simulink model "SYDE_351_Project"  (R2022b)
settings: Solver=VariableStepAuto  StartTime=0.0  StopTime=23.55  RelTol=1e-3
values from neighbouring files (symbols this model uses):
  d = 2.5e-2    (= 0.025)    [SYDE_351_Project_Parameters.m]
  J = (1/2)*(M * (R_cyl)^2)    (= 0.625)    [SYDE_351_Project_Parameters.m]
  K_b = 0.3247    [SYDE_351_Project_Parameters.m]
  K_t = 0.3248    [SYDE_351_Project_Parameters.m]
  L = 25e-2    (= 0.25)    [SYDE_351_Project_Parameters.m]
  L_a = 6.6e-3    (= 0.0066)    [SYDE_351_Project_Parameters.m]
  M = 20    [SYDE_351_Project_Parameters.m]
  N = 1    [SYDE_351_Project_Parameters.m]
  R = 5e-2    (= 0.05)    [SYDE_351_Project_Parameters.m]
  R_a = 4    [SYDE_351_Project_Parameters.m]
libraries: slpidlib x6
settings Model: Creator=danielkang  LastModifiedBy=danielkang

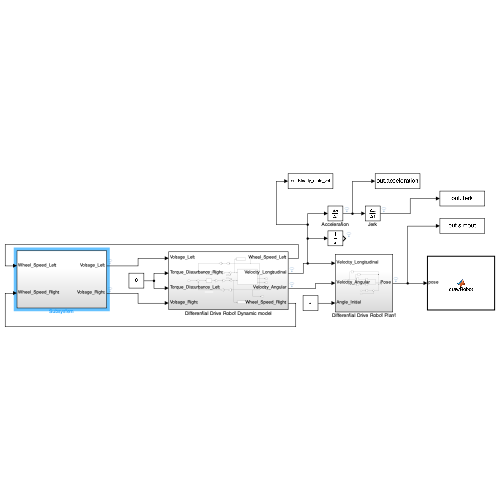
[thumbnail: Simulink's stored preview of the top-level diagram]
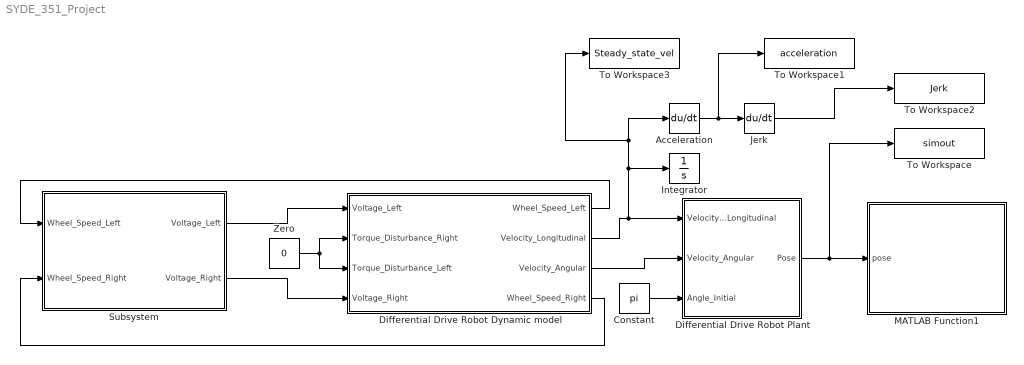
== system SYDE_351_Project ==
  Acceleration : Derivative
  Constant : Constant  Value=pi
  Differential Drive Robot Dynamic model : Subsystem
  Differential Drive Robot Plant : Subsystem
  Integrator : Integrator
  Jerk : Derivative
  MATLAB Function1 : MATLAB Function  TreatAsAtomicUnit=on
  Subsystem : Subsystem
  To Workspace : ToWorkspace  VariableName=simout  SampleTime=-1
      settings: Save2DSignal=2-D array (concatenate along first dimension)
  To Workspace1 : ToWorkspace  VariableName=acceleration  SampleTime=-1
      settings: Save2DSignal=2-D array (concatenate along first dimension)
  To Workspace2 : ToWorkspace  VariableName=Jerk  SampleTime=-1
      settings: Save2DSignal=2-D array (concatenate along first dimension)
  To Workspace3 : ToWorkspace  VariableName=Steady_state_vel  SampleTime=-1
      settings: Save2DSignal=2-D array (concatenate along first dimension)
  Zero : Constant  Value=0  OutDataTypeStr=Inherit: Inherit via back propagation
  wires:
  Zero/1 -> Differential Drive Robot Dynamic model/3(Torque_Disturbance_Left), Differential Drive Robot Dynamic model/2(Torque_Disturbance_Right)
  Differential Drive Robot Dynamic model/3(Velocity_Angular) -> Differential Drive Robot Plant/2(Velocity_Angular)
  Differential Drive Robot Plant/1(Pose) -> To Workspace/1, MATLAB Function1/1(pose)
  Differential Drive Robot Dynamic model/2(Velocity_Longitudinal) -> Integrator/1, To Workspace3/1, Acceleration/1, Differential Drive Robot Plant/1(Velocity_Longitudinal)
  Constant/1 -> Differential Drive Robot Plant/3(Angle_Initial)
  Acceleration/1 -> To Workspace1/1, Jerk/1
  Jerk/1 -> To Workspace2/1
  Subsystem/1(Voltage_Left) -> Differential Drive Robot Dynamic model/1(Voltage_Left)
  Subsystem/2(Voltage_Right) -> Differential Drive Robot Dynamic model/4(Voltage_Right)
  Differential Drive Robot Dynamic model/1(Wheel_Speed_Left) -> Subsystem/1(Wheel_Speed_Left)
  Differential Drive Robot Dynamic model/4(Wheel_Speed_Right) -> Subsystem/2(Wheel_Speed_Right)

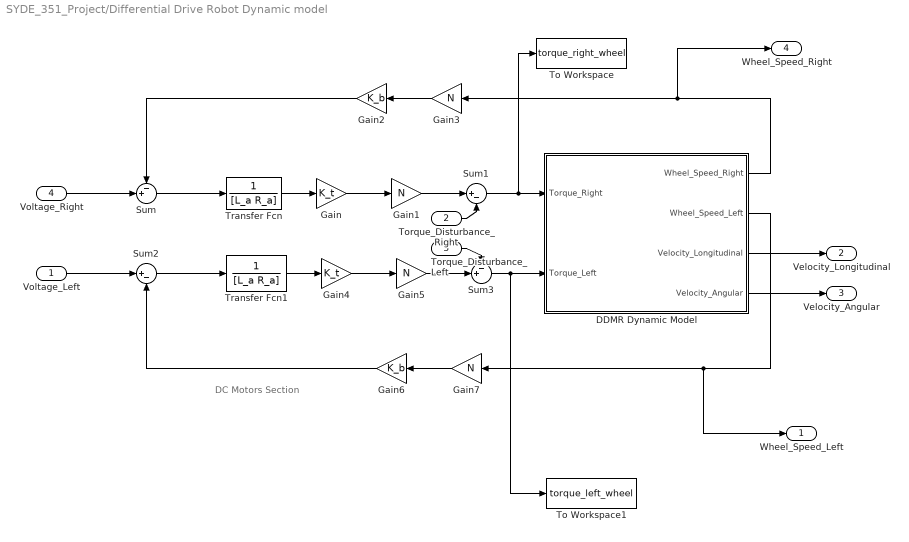
== system SYDE_351_Project/Differential Drive Robot Dynamic model ==
  note: DC Motors Section
  Voltage_Left : Inport
  Torque_Disturbance_Right : Inport  Port=2
  Torque_Disturbance_Left : Inport  Port=3
  Voltage_Right : Inport  Port=4
  DDMR Dynamic Model : Subsystem
  Gain : Gain  Gain=K_t
  Gain{1,3,5,7} (4 alike) : Gain  Gain=N
  Gain2 : Gain  Gain=K_b
  Gain4 : Gain  Gain=K_t
  Gain6 : Gain  Gain=K_b
  Sum : Sum  Inputs=-+|
  Sum1 : Sum  Inputs=|+-
  Sum2 : Sum  Inputs=|+-
  Sum3 : Sum  Inputs=-+|
  To Workspace : ToWorkspace  VariableName=torque_right_wheel  SaveFormat=Structure With Time  SampleTime=-1
      settings: Save2DSignal=2-D array (concatenate along first dimension)
  To Workspace1 : ToWorkspace  VariableName=torque_left_wheel  SaveFormat=Structure With Time  SampleTime=-1
  Transfer Fcn : TransferFcn  Denominator=[L_a R_a]
  Transfer Fcn1 : TransferFcn  Denominator=[L_a R_a]
  Wheel_Speed_Left : Outport
  Velocity_Longitudinal : Outport  Port=2
  Velocity_Angular : Outport  Port=3
  Wheel_Speed_Right : Outport  Port=4
  wires:
  Torque_Disturbance_Left/1 -> Sum3/1
  Gain5/1 -> Sum3/2
  Torque_Disturbance_Right/1 -> Sum1/2
  Gain7/1 -> Gain6/1
  Sum/1 -> Transfer Fcn/1
  Transfer Fcn1/1 -> Gain4/1
  Sum3/1 -> To Workspace1/1, DDMR Dynamic Model/2(Torque_Left)
  Sum1/1 -> To Workspace/1, DDMR Dynamic Model/1(Torque_Right)
  Gain6/1 -> Sum2/2
  Gain3/1 -> Gain2/1
  Sum2/1 -> Transfer Fcn1/1
  Gain4/1 -> Gain5/1
  Voltage_Right/1 -> Sum/2
  Voltage_Left/1 -> Sum2/1
  Gain2/1 -> Sum/1
  Transfer Fcn/1 -> Gain/1
  Gain/1 -> Gain1/1
  Gain1/1 -> Sum1/1
  DDMR Dynamic Model/1(Wheel_Speed_Right) -> Wheel_Speed_Right/1, Gain3/1
  DDMR Dynamic Model/3(Velocity_Longitudinal) -> Velocity_Longitudinal/1
  DDMR Dynamic Model/4(Velocity_Angular) -> Velocity_Angular/1
  DDMR Dynamic Model/2(Wheel_Speed_Left) -> Wheel_Speed_Left/1, Gain7/1

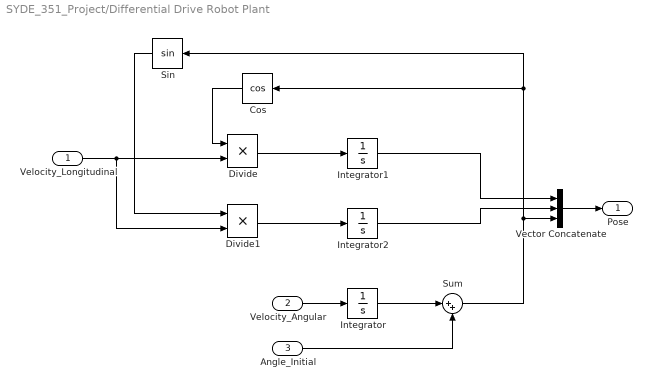
== system SYDE_351_Project/Differential Drive Robot Plant ==
  Velocity_Longitudinal : Inport
  Velocity_Angular : Inport  Port=2
  Angle_Initial : Inport  Port=3
  Cos : Trigonometry  Operator=cos
  Divide : Product  Inputs=**
  Divide1 : Product  Inputs=**
  Integrator : Integrator
  Integrator1 : Integrator
  Integrator2 : Integrator
  Sin : Trigonometry
  Sum : Sum  Inputs=|++
  Vector Concatenate : Concatenate  NumInputs=3
  Pose : Outport
  wires:
  Velocity_Angular/1 -> Integrator/1
  Cos/1 -> Divide/1
  Divide/1 -> Integrator1/1
  Integrator1/1 -> Vector Concatenate/1
  Velocity_Longitudinal/1 -> Divide1/2, Divide/2
  Divide1/1 -> Integrator2/1
  Integrator2/1 -> Vector Concatenate/2
  Sin/1 -> Divide1/1
  Vector Concatenate/1 -> Pose/1
  Angle_Initial/1 -> Sum/2
  Integrator/1 -> Sum/1
  Sum/1 -> Cos/1, Sin/1, Vector Concatenate/3

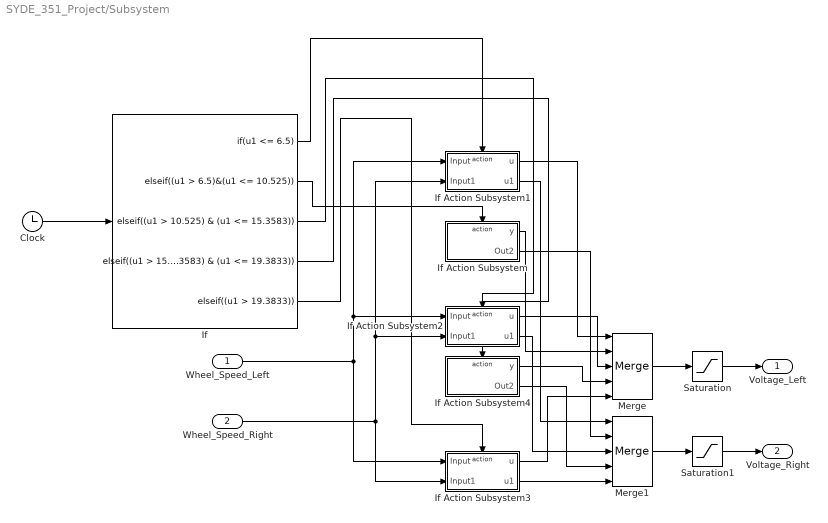
== system SYDE_351_Project/Subsystem ==
  Wheel_Speed_Left : Inport
  Wheel_Speed_Right : Inport  Port=2
  Clock : Clock
  If : If  IfExpression=u1 <= 6.5  ElseIfExpressions=(u1 > 6.5)&(u1 <= 10.525), (u1 > 10.525) & (u1 <= 15.3583), (u1 > 15.3583) & (u1 <= 19.3833),(u1 > 19.3833)  ShowElse=off
  If Action Subsystem : Subsystem  TreatAsAtomicUnit=on
  If Action Subsystem1 : Subsystem  TreatAsAtomicUnit=on
  If Action Subsystem2 : Subsystem  TreatAsAtomicUnit=on
  If Action Subsystem3 : Subsystem  TreatAsAtomicUnit=on
  If Action Subsystem4 : Subsystem  TreatAsAtomicUnit=on
  Merge : Merge  Inputs=5
  Merge1 : Merge  Inputs=5
  Saturation : Saturate  UpperLimit=500  LowerLimit=-500
  Saturation1 : Saturate  UpperLimit=500  LowerLimit=-500
  Voltage_Left : Outport
  Voltage_Right : Outport  Port=2
  wires:
  If Action Subsystem2/2(u1) -> Merge1/3
  If Action Subsystem2/1(u) -> Merge/3
  If Action Subsystem1/1(u) -> Merge/1
  If/1 -> If Action Subsystem1/Action
  If Action Subsystem1/2(u1) -> Merge1/1
  Clock/1 -> If/1
  Wheel_Speed_Left/1 -> If Action Subsystem1/1(Input), If Action Subsystem2/1(Input), If Action Subsystem3/1(Input)
  Wheel_Speed_Right/1 -> If Action Subsystem1/2(Input1), If Action Subsystem2/2(Input1), If Action Subsystem3/2(Input1)
  If/2 -> If Action Subsystem/Action
  If Action Subsystem/1(y) -> Merge/2
  If Action Subsystem/2(Out2) -> Merge1/2
  If/3 -> If Action Subsystem2/Action
  Saturation/1 -> Voltage_Left/1
  Merge/1 -> Saturation/1
  Merge1/1 -> Saturation1/1
  Saturation1/1 -> Voltage_Right/1
  If/4 -> If Action Subsystem4/Action
  If/5 -> If Action Subsystem3/Action
  If Action Subsystem4/1(y) -> Merge/4
  If Action Subsystem4/2(Out2) -> Merge1/4
  If Action Subsystem3/1(u) -> Merge/5
  If Action Subsystem3/2(u1) -> Merge1/5

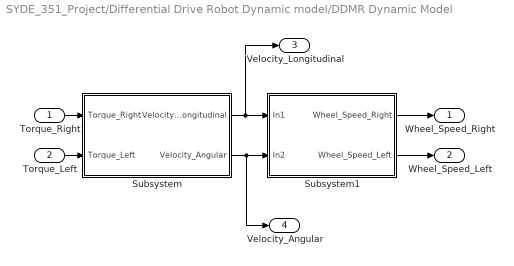
== system SYDE_351_Project/Differential Drive Robot Dynamic model/DDMR Dynamic Model ==
  Torque_Right : Inport
  Torque_Left : Inport  Port=2
  Subsystem : Subsystem
  Subsystem1 : Subsystem
  Wheel_Speed_Right : Outport
  Wheel_Speed_Left : Outport  Port=2
  Velocity_Longitudinal : Outport  Port=3
  Velocity_Angular : Outport  Port=4
  wires:
  Torque_Right/1 -> Subsystem/1(Torque_Right)
  Subsystem/1(Velocity_Longitudinal) -> Velocity_Longitudinal/1, Subsystem1/1(In1)
  Subsystem1/1(Wheel_Speed_Right) -> Wheel_Speed_Right/1
  Subsystem1/2(Wheel_Speed_Left) -> Wheel_Speed_Left/1
  Torque_Left/1 -> Subsystem/2(Torque_Left)
  Subsystem/2(Velocity_Angular) -> Velocity_Angular/1, Subsystem1/2(In2)

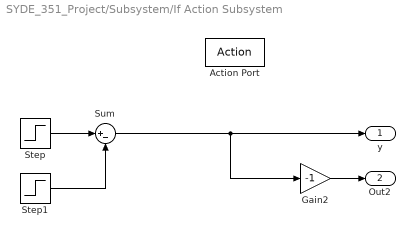
== system SYDE_351_Project/Subsystem/If Action Subsystem ==
  Action Port : ActionPort  ActionPortLabel=elseif((u1 > 6.5)&(u1 <= 10.525))
  Gain2 : Gain  Gain=-1
  Step : Step  Time=6.5  After=2  SampleTime=0
  Step1 : Step  Time=7.77  After=2  SampleTime=0
  Sum : Sum  Inputs=|+-
  y : Outport
  Out2 : Outport  Port=2
  wires:
  Gain2/1 -> Out2/1
  Sum/1 -> y/1, Gain2/1
  Step/1 -> Sum/1
  Step1/1 -> Sum/2

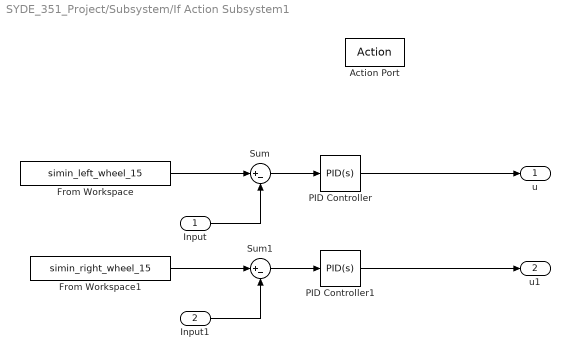
== system SYDE_351_Project/Subsystem/If Action Subsystem1 ==
  Input : Inport
  Input1 : Inport  Port=2
  Action Port : ActionPort  ActionPortLabel=if(u1 <= 6.5)
  From Workspace : FromWorkspace  VariableName=simin_left_wheel_15  ZeroCross=off
  From Workspace1 : FromWorkspace  VariableName=simin_right_wheel_15  ZeroCross=off
  PID Controller : slpidlib/PID Controller  Controller=PID  Form=Parallel  TimeDomain=Continuous-time  UseExternalTs=off  SampleTime=-1  IntegratorMethod=Forward Euler  FilterMethod=Forward Euler  ControllerParametersSource=internal  P=50  I=0  UseKiTs=off  D=0  N=100  UseFilter=on  TunerSelectOption=Transfer Function Based (PID Tuner App)  InitialConditionSource=internal  InitialConditionForIntegrator=0  InitialConditionForFilter=0  DifferentiatorICPrevScaledInput=0  ExternalReset=none  TrackingMode=off  Kt=1  LimitOutput=off  SatLimitsSource=internal  UpperSaturationLimit=inf  LowerSaturationLimit=-inf  LinearizeAsGain=on  AntiWindupMode=none  Kb=1  LimitIntegrator=off  UpperIntegratorSaturationLimit=inf  LowerIntegratorSaturationLimit=-inf  POutMin=[]  POutMax=[]  IOutMin=[]  IOutMax=[]  DOutMin=[]  DOutMax=[]  NOutMin=[]  NOutMax=[]  SumOutMin=[]  SumOutMax=[]  SaturationOutMin=[]  SaturationOutMax=[]  PParamMin=[]  PParamMax=[]  IParamMin=[]  IParamMax=[]  DParamMin=[]  DParamMax=[]  NParamMin=[]  NParamMax=[]  KbParamMin=[]  KbParamMax=[]  KtParamMin=[]  KtParamMax=[]  KbOutMin=[]  KbOutMax=[]  KtOutMin=[]  KtOutMax=[]  IntegratorOutMin=[]  IntegratorOutMax=[]  FilterOutMin=[]  FilterOutMax=[]  SumI1OutMin=[]  SumI1OutMax=[]  SumI2OutMin=[]  SumI2OutMax=[]  SumI3OutMin=[]  SumI3OutMax=[]  SumI4OutMin=[]  SumI4OutMax=[]  SumDOutMin=[]  SumDOutMax=[]  DifferentiatorOutMin=[]  DifferentiatorOutMax=[]  FilterDiffOutCoefMin=[]  FilterDiffOutCoefMax=[]  ReciprocalOutMin=[]  ReciprocalOutMax=[]  SumDenOutMin=[]  SumDenOutMax=[]  SumNumOutMin=[]  SumNumOutMax=[]  DivideOutMin=[]  DivideOutMax=[]  UdiffTsProdOutMin=[]  UdiffTsProdOutMax=[]  NTsProdOutMin=[]  NTsProdOutMax=[]  UintegralTsProdOutMin=[]  UintegralTsProdOutMax=[]  UngainTsProdOutMin=[]  UngainTsProdOutMax=[]  ClampingZeroOutDataTypeStr=Inherit: Inherit via back propagation  ClampingZeroOutMin=[]  ClampingZeroOutMax=[]  FilterDenConstantOutDataTypeStr=Inherit: Inherit via back propagation  FilterDenConstantOutMin=[]  FilterDenConstantOutMax=[]  PCopyOutDataTypeStr=Inherit: Inherit via back propagation  PCopyOutMin=[]  PCopyOutMax=[]  NCopyOutDataTypeStr=Inherit: Inherit via back propagation  NCopyOutMin=[]  NCopyOutMax=[]  IntegratorContinuousStateAttributes=''  IntegratorStateMustResolveToSignalObject=off  IntegratorRTWStateStorageClass=Auto  FilterContinuousStateAttributes=''  FilterStateMustResolveToSignalObject=off  FilterRTWStateStorageClass=Auto  ParallelPVariant=InternalParameters  IdealPVariant=Disabled  IVariant=InternalParameters  DVariant=InternalParameters  IntegratorVariant=Continuous  SatVariant=Disabled  AWVariant=Passthrough  PCopyVariant=Disabled  TRVariant=Disabled  FdbkBlocksVariant=Forward  IdealPFdbkVariant=Disabled  SatFdbkVariant=Disabled  DerivativeFilterVariant=ContFilter  NVariant=InternalParameters  NCopyVariant=Disabled  FilterICVariant=InternalICsFilter  IntegratorICVariant=InternalICs  ExternalResetVariant=Disabled  TRSumVariant=Passthrough  SumFdbkVariant=Disabled  SumVariant=Sum_PID  TsampFilterVariant=InternalTs  TsampNgainVariant=Passthrough  TsampIntegralVariant=Passthrough  ExternalSaturationOutDataTypeStr=Inherit: Same as second input
  PID Controller1 : slpidlib/PID Controller  Controller=PID  Form=Parallel  TimeDomain=Continuous-time  UseExternalTs=off  SampleTime=-1  IntegratorMethod=Forward Euler  FilterMethod=Forward Euler  ControllerParametersSource=internal  P=50  I=0  UseKiTs=off  D=0  N=100  UseFilter=on  TunerSelectOption=Transfer Function Based (PID Tuner App)  InitialConditionSource=internal  InitialConditionForIntegrator=0  InitialConditionForFilter=0  DifferentiatorICPrevScaledInput=0  ExternalReset=none  TrackingMode=off  Kt=1  LimitOutput=off  SatLimitsSource=internal  UpperSaturationLimit=inf  LowerSaturationLimit=-inf  LinearizeAsGain=on  AntiWindupMode=none  Kb=1  LimitIntegrator=off  UpperIntegratorSaturationLimit=inf  LowerIntegratorSaturationLimit=-inf  POutMin=[]  POutMax=[]  IOutMin=[]  IOutMax=[]  DOutMin=[]  DOutMax=[]  NOutMin=[]  NOutMax=[]  SumOutMin=[]  SumOutMax=[]  SaturationOutMin=[]  SaturationOutMax=[]  PParamMin=[]  PParamMax=[]  IParamMin=[]  IParamMax=[]  DParamMin=[]  DParamMax=[]  NParamMin=[]  NParamMax=[]  KbParamMin=[]  KbParamMax=[]  KtParamMin=[]  KtParamMax=[]  KbOutMin=[]  KbOutMax=[]  KtOutMin=[]  KtOutMax=[]  IntegratorOutMin=[]  IntegratorOutMax=[]  FilterOutMin=[]  FilterOutMax=[]  SumI1OutMin=[]  SumI1OutMax=[]  SumI2OutMin=[]  SumI2OutMax=[]  SumI3OutMin=[]  SumI3OutMax=[]  SumI4OutMin=[]  SumI4OutMax=[]  SumDOutMin=[]  SumDOutMax=[]  DifferentiatorOutMin=[]  DifferentiatorOutMax=[]  FilterDiffOutCoefMin=[]  FilterDiffOutCoefMax=[]  ReciprocalOutMin=[]  ReciprocalOutMax=[]  SumDenOutMin=[]  SumDenOutMax=[]  SumNumOutMin=[]  SumNumOutMax=[]  DivideOutMin=[]  DivideOutMax=[]  UdiffTsProdOutMin=[]  UdiffTsProdOutMax=[]  NTsProdOutMin=[]  NTsProdOutMax=[]  UintegralTsProdOutMin=[]  UintegralTsProdOutMax=[]  UngainTsProdOutMin=[]  UngainTsProdOutMax=[]  ClampingZeroOutDataTypeStr=Inherit: Inherit via back propagation  ClampingZeroOutMin=[]  ClampingZeroOutMax=[]  FilterDenConstantOutDataTypeStr=Inherit: Inherit via back propagation  FilterDenConstantOutMin=[]  FilterDenConstantOutMax=[]  PCopyOutDataTypeStr=Inherit: Inherit via back propagation  PCopyOutMin=[]  PCopyOutMax=[]  NCopyOutDataTypeStr=Inherit: Inherit via back propagation  NCopyOutMin=[]  NCopyOutMax=[]  IntegratorContinuousStateAttributes=''  IntegratorStateMustResolveToSignalObject=off  IntegratorRTWStateStorageClass=Auto  FilterContinuousStateAttributes=''  FilterStateMustResolveToSignalObject=off  FilterRTWStateStorageClass=Auto  ParallelPVariant=InternalParameters  IdealPVariant=Disabled  IVariant=InternalParameters  DVariant=InternalParameters  IntegratorVariant=Continuous  SatVariant=Disabled  AWVariant=Passthrough  PCopyVariant=Disabled  TRVariant=Disabled  FdbkBlocksVariant=Forward  IdealPFdbkVariant=Disabled  SatFdbkVariant=Disabled  DerivativeFilterVariant=ContFilter  NVariant=InternalParameters  NCopyVariant=Disabled  FilterICVariant=InternalICsFilter  IntegratorICVariant=InternalICs  ExternalResetVariant=Disabled  TRSumVariant=Passthrough  SumFdbkVariant=Disabled  SumVariant=Sum_PID  TsampFilterVariant=InternalTs  TsampNgainVariant=Passthrough  TsampIntegralVariant=Passthrough  ExternalSaturationOutDataTypeStr=Inherit: Same as second input
  Sum : Sum  Inputs=|+-
  Sum1 : Sum  Inputs=|+-
  u : Outport
  u1 : Outport  Port=2
  wires:
  Sum1/1 -> PID Controller1/1
  Input1/1 -> Sum1/2
  Sum/1 -> PID Controller/1
  PID Controller1/1 -> u1/1
  Input/1 -> Sum/2
  PID Controller/1 -> u/1
  From Workspace1/1 -> Sum1/1
  From Workspace/1 -> Sum/1

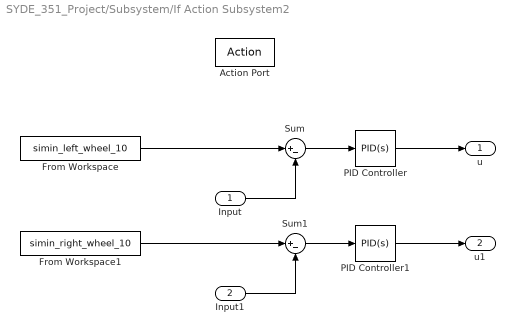
== system SYDE_351_Project/Subsystem/If Action Subsystem2 ==
  Input : Inport
  Input1 : Inport  Port=2
  Action Port : ActionPort  ActionPortLabel=elseif( (u1 > 10.525) & (u1 <= 15.3583))
  From Workspace : FromWorkspace  VariableName=simin_left_wheel_10  ZeroCross=off
  From Workspace1 : FromWorkspace  VariableName=simin_right_wheel_10  ZeroCross=off
  PID Controller : slpidlib/PID Controller  Controller=PID  Form=Parallel  TimeDomain=Continuous-time  UseExternalTs=off  SampleTime=-1  IntegratorMethod=Forward Euler  FilterMethod=Forward Euler  ControllerParametersSource=internal  P=50  I=0  UseKiTs=off  D=0  N=100  UseFilter=on  TunerSelectOption=Transfer Function Based (PID Tuner App)  InitialConditionSource=internal  InitialConditionForIntegrator=0  InitialConditionForFilter=0  DifferentiatorICPrevScaledInput=0  ExternalReset=none  TrackingMode=off  Kt=1  LimitOutput=off  SatLimitsSource=internal  UpperSaturationLimit=inf  LowerSaturationLimit=-inf  LinearizeAsGain=on  AntiWindupMode=none  Kb=1  LimitIntegrator=off  UpperIntegratorSaturationLimit=inf  LowerIntegratorSaturationLimit=-inf  POutMin=[]  POutMax=[]  IOutMin=[]  IOutMax=[]  DOutMin=[]  DOutMax=[]  NOutMin=[]  NOutMax=[]  SumOutMin=[]  SumOutMax=[]  SaturationOutMin=[]  SaturationOutMax=[]  PParamMin=[]  PParamMax=[]  IParamMin=[]  IParamMax=[]  DParamMin=[]  DParamMax=[]  NParamMin=[]  NParamMax=[]  KbParamMin=[]  KbParamMax=[]  KtParamMin=[]  KtParamMax=[]  KbOutMin=[]  KbOutMax=[]  KtOutMin=[]  KtOutMax=[]  IntegratorOutMin=[]  IntegratorOutMax=[]  FilterOutMin=[]  FilterOutMax=[]  SumI1OutMin=[]  SumI1OutMax=[]  SumI2OutMin=[]  SumI2OutMax=[]  SumI3OutMin=[]  SumI3OutMax=[]  SumI4OutMin=[]  SumI4OutMax=[]  SumDOutMin=[]  SumDOutMax=[]  DifferentiatorOutMin=[]  DifferentiatorOutMax=[]  FilterDiffOutCoefMin=[]  FilterDiffOutCoefMax=[]  ReciprocalOutMin=[]  ReciprocalOutMax=[]  SumDenOutMin=[]  SumDenOutMax=[]  SumNumOutMin=[]  SumNumOutMax=[]  DivideOutMin=[]  DivideOutMax=[]  UdiffTsProdOutMin=[]  UdiffTsProdOutMax=[]  NTsProdOutMin=[]  NTsProdOutMax=[]  UintegralTsProdOutMin=[]  UintegralTsProdOutMax=[]  UngainTsProdOutMin=[]  UngainTsProdOutMax=[]  ClampingZeroOutDataTypeStr=Inherit: Inherit via back propagation  ClampingZeroOutMin=[]  ClampingZeroOutMax=[]  FilterDenConstantOutDataTypeStr=Inherit: Inherit via back propagation  FilterDenConstantOutMin=[]  FilterDenConstantOutMax=[]  PCopyOutDataTypeStr=Inherit: Inherit via back propagation  PCopyOutMin=[]  PCopyOutMax=[]  NCopyOutDataTypeStr=Inherit: Inherit via back propagation  NCopyOutMin=[]  NCopyOutMax=[]  IntegratorContinuousStateAttributes=''  IntegratorStateMustResolveToSignalObject=off  IntegratorRTWStateStorageClass=Auto  FilterContinuousStateAttributes=''  FilterStateMustResolveToSignalObject=off  FilterRTWStateStorageClass=Auto  ParallelPVariant=InternalParameters  IdealPVariant=Disabled  IVariant=InternalParameters  DVariant=InternalParameters  IntegratorVariant=Continuous  SatVariant=Disabled  AWVariant=Passthrough  PCopyVariant=Disabled  TRVariant=Disabled  FdbkBlocksVariant=Forward  IdealPFdbkVariant=Disabled  SatFdbkVariant=Disabled  DerivativeFilterVariant=ContFilter  NVariant=InternalParameters  NCopyVariant=Disabled  FilterICVariant=InternalICsFilter  IntegratorICVariant=InternalICs  ExternalResetVariant=Disabled  TRSumVariant=Passthrough  SumFdbkVariant=Disabled  SumVariant=Sum_PID  TsampFilterVariant=InternalTs  TsampNgainVariant=Passthrough  TsampIntegralVariant=Passthrough  ExternalSaturationOutDataTypeStr=Inherit: Same as second input
  PID Controller1 : slpidlib/PID Controller  Controller=PID  Form=Parallel  TimeDomain=Continuous-time  UseExternalTs=off  SampleTime=-1  IntegratorMethod=Forward Euler  FilterMethod=Forward Euler  ControllerParametersSource=internal  P=50  I=0  UseKiTs=off  D=0  N=100  UseFilter=on  TunerSelectOption=Transfer Function Based (PID Tuner App)  InitialConditionSource=internal  InitialConditionForIntegrator=0  InitialConditionForFilter=0  DifferentiatorICPrevScaledInput=0  ExternalReset=none  TrackingMode=off  Kt=1  LimitOutput=off  SatLimitsSource=internal  UpperSaturationLimit=inf  LowerSaturationLimit=-inf  LinearizeAsGain=on  AntiWindupMode=none  Kb=1  LimitIntegrator=off  UpperIntegratorSaturationLimit=inf  LowerIntegratorSaturationLimit=-inf  POutMin=[]  POutMax=[]  IOutMin=[]  IOutMax=[]  DOutMin=[]  DOutMax=[]  NOutMin=[]  NOutMax=[]  SumOutMin=[]  SumOutMax=[]  SaturationOutMin=[]  SaturationOutMax=[]  PParamMin=[]  PParamMax=[]  IParamMin=[]  IParamMax=[]  DParamMin=[]  DParamMax=[]  NParamMin=[]  NParamMax=[]  KbParamMin=[]  KbParamMax=[]  KtParamMin=[]  KtParamMax=[]  KbOutMin=[]  KbOutMax=[]  KtOutMin=[]  KtOutMax=[]  IntegratorOutMin=[]  IntegratorOutMax=[]  FilterOutMin=[]  FilterOutMax=[]  SumI1OutMin=[]  SumI1OutMax=[]  SumI2OutMin=[]  SumI2OutMax=[]  SumI3OutMin=[]  SumI3OutMax=[]  SumI4OutMin=[]  SumI4OutMax=[]  SumDOutMin=[]  SumDOutMax=[]  DifferentiatorOutMin=[]  DifferentiatorOutMax=[]  FilterDiffOutCoefMin=[]  FilterDiffOutCoefMax=[]  ReciprocalOutMin=[]  ReciprocalOutMax=[]  SumDenOutMin=[]  SumDenOutMax=[]  SumNumOutMin=[]  SumNumOutMax=[]  DivideOutMin=[]  DivideOutMax=[]  UdiffTsProdOutMin=[]  UdiffTsProdOutMax=[]  NTsProdOutMin=[]  NTsProdOutMax=[]  UintegralTsProdOutMin=[]  UintegralTsProdOutMax=[]  UngainTsProdOutMin=[]  UngainTsProdOutMax=[]  ClampingZeroOutDataTypeStr=Inherit: Inherit via back propagation  ClampingZeroOutMin=[]  ClampingZeroOutMax=[]  FilterDenConstantOutDataTypeStr=Inherit: Inherit via back propagation  FilterDenConstantOutMin=[]  FilterDenConstantOutMax=[]  PCopyOutDataTypeStr=Inherit: Inherit via back propagation  PCopyOutMin=[]  PCopyOutMax=[]  NCopyOutDataTypeStr=Inherit: Inherit via back propagation  NCopyOutMin=[]  NCopyOutMax=[]  IntegratorContinuousStateAttributes=''  IntegratorStateMustResolveToSignalObject=off  IntegratorRTWStateStorageClass=Auto  FilterContinuousStateAttributes=''  FilterStateMustResolveToSignalObject=off  FilterRTWStateStorageClass=Auto  ParallelPVariant=InternalParameters  IdealPVariant=Disabled  IVariant=InternalParameters  DVariant=InternalParameters  IntegratorVariant=Continuous  SatVariant=Disabled  AWVariant=Passthrough  PCopyVariant=Disabled  TRVariant=Disabled  FdbkBlocksVariant=Forward  IdealPFdbkVariant=Disabled  SatFdbkVariant=Disabled  DerivativeFilterVariant=ContFilter  NVariant=InternalParameters  NCopyVariant=Disabled  FilterICVariant=InternalICsFilter  IntegratorICVariant=InternalICs  ExternalResetVariant=Disabled  TRSumVariant=Passthrough  SumFdbkVariant=Disabled  SumVariant=Sum_PID  TsampFilterVariant=InternalTs  TsampNgainVariant=Passthrough  TsampIntegralVariant=Passthrough  ExternalSaturationOutDataTypeStr=Inherit: Same as second input
  Sum : Sum  Inputs=|+-
  Sum1 : Sum  Inputs=|+-
  u : Outport
  u1 : Outport  Port=2
  wires:
  Sum1/1 -> PID Controller1/1
  Input1/1 -> Sum1/2
  Sum/1 -> PID Controller/1
  Input/1 -> Sum/2
  From Workspace1/1 -> Sum1/1
  From Workspace/1 -> Sum/1
  PID Controller/1 -> u/1
  PID Controller1/1 -> u1/1

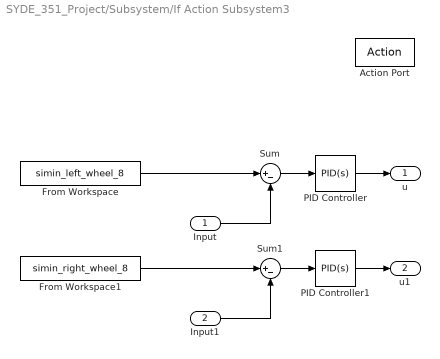
== system SYDE_351_Project/Subsystem/If Action Subsystem3 ==
  Input : Inport
  Input1 : Inport  Port=2
  Action Port : ActionPort  ActionPortLabel=elseif((u1 > 19.3833))
  From Workspace : FromWorkspace  VariableName=simin_left_wheel_8  ZeroCross=off
  From Workspace1 : FromWorkspace  VariableName=simin_right_wheel_8  ZeroCross=off
  PID Controller : slpidlib/PID Controller  Controller=PID  Form=Parallel  TimeDomain=Continuous-time  UseExternalTs=off  SampleTime=-1  IntegratorMethod=Forward Euler  FilterMethod=Forward Euler  ControllerParametersSource=internal  P=50  I=0  UseKiTs=off  D=0  N=100  UseFilter=on  TunerSelectOption=Transfer Function Based (PID Tuner App)  InitialConditionSource=internal  InitialConditionForIntegrator=0  InitialConditionForFilter=0  DifferentiatorICPrevScaledInput=0  ExternalReset=none  TrackingMode=off  Kt=1  LimitOutput=off  SatLimitsSource=internal  UpperSaturationLimit=inf  LowerSaturationLimit=-inf  LinearizeAsGain=on  AntiWindupMode=none  Kb=1  LimitIntegrator=off  UpperIntegratorSaturationLimit=inf  LowerIntegratorSaturationLimit=-inf  POutMin=[]  POutMax=[]  IOutMin=[]  IOutMax=[]  DOutMin=[]  DOutMax=[]  NOutMin=[]  NOutMax=[]  SumOutMin=[]  SumOutMax=[]  SaturationOutMin=[]  SaturationOutMax=[]  PParamMin=[]  PParamMax=[]  IParamMin=[]  IParamMax=[]  DParamMin=[]  DParamMax=[]  NParamMin=[]  NParamMax=[]  KbParamMin=[]  KbParamMax=[]  KtParamMin=[]  KtParamMax=[]  KbOutMin=[]  KbOutMax=[]  KtOutMin=[]  KtOutMax=[]  IntegratorOutMin=[]  IntegratorOutMax=[]  FilterOutMin=[]  FilterOutMax=[]  SumI1OutMin=[]  SumI1OutMax=[]  SumI2OutMin=[]  SumI2OutMax=[]  SumI3OutMin=[]  SumI3OutMax=[]  SumI4OutMin=[]  SumI4OutMax=[]  SumDOutMin=[]  SumDOutMax=[]  DifferentiatorOutMin=[]  DifferentiatorOutMax=[]  FilterDiffOutCoefMin=[]  FilterDiffOutCoefMax=[]  ReciprocalOutMin=[]  ReciprocalOutMax=[]  SumDenOutMin=[]  SumDenOutMax=[]  SumNumOutMin=[]  SumNumOutMax=[]  DivideOutMin=[]  DivideOutMax=[]  UdiffTsProdOutMin=[]  UdiffTsProdOutMax=[]  NTsProdOutMin=[]  NTsProdOutMax=[]  UintegralTsProdOutMin=[]  UintegralTsProdOutMax=[]  UngainTsProdOutMin=[]  UngainTsProdOutMax=[]  ClampingZeroOutDataTypeStr=Inherit: Inherit via back propagation  ClampingZeroOutMin=[]  ClampingZeroOutMax=[]  FilterDenConstantOutDataTypeStr=Inherit: Inherit via back propagation  FilterDenConstantOutMin=[]  FilterDenConstantOutMax=[]  PCopyOutDataTypeStr=Inherit: Inherit via back propagation  PCopyOutMin=[]  PCopyOutMax=[]  NCopyOutDataTypeStr=Inherit: Inherit via back propagation  NCopyOutMin=[]  NCopyOutMax=[]  IntegratorContinuousStateAttributes=''  IntegratorStateMustResolveToSignalObject=off  IntegratorRTWStateStorageClass=Auto  FilterContinuousStateAttributes=''  FilterStateMustResolveToSignalObject=off  FilterRTWStateStorageClass=Auto  ParallelPVariant=InternalParameters  IdealPVariant=Disabled  IVariant=InternalParameters  DVariant=InternalParameters  IntegratorVariant=Continuous  SatVariant=Disabled  AWVariant=Passthrough  PCopyVariant=Disabled  TRVariant=Disabled  FdbkBlocksVariant=Forward  IdealPFdbkVariant=Disabled  SatFdbkVariant=Disabled  DerivativeFilterVariant=ContFilter  NVariant=InternalParameters  NCopyVariant=Disabled  FilterICVariant=InternalICsFilter  IntegratorICVariant=InternalICs  ExternalResetVariant=Disabled  TRSumVariant=Passthrough  SumFdbkVariant=Disabled  SumVariant=Sum_PID  TsampFilterVariant=InternalTs  TsampNgainVariant=Passthrough  TsampIntegralVariant=Passthrough  ExternalSaturationOutDataTypeStr=Inherit: Same as second input
  PID Controller1 : slpidlib/PID Controller  Controller=PID  Form=Parallel  TimeDomain=Continuous-time  UseExternalTs=off  SampleTime=-1  IntegratorMethod=Forward Euler  FilterMethod=Forward Euler  ControllerParametersSource=internal  P=50  I=0  UseKiTs=off  D=0  N=100  UseFilter=on  TunerSelectOption=Transfer Function Based (PID Tuner App)  InitialConditionSource=internal  InitialConditionForIntegrator=0  InitialConditionForFilter=0  DifferentiatorICPrevScaledInput=0  ExternalReset=none  TrackingMode=off  Kt=1  LimitOutput=off  SatLimitsSource=internal  UpperSaturationLimit=inf  LowerSaturationLimit=-inf  LinearizeAsGain=on  AntiWindupMode=none  Kb=1  LimitIntegrator=off  UpperIntegratorSaturationLimit=inf  LowerIntegratorSaturationLimit=-inf  POutMin=[]  POutMax=[]  IOutMin=[]  IOutMax=[]  DOutMin=[]  DOutMax=[]  NOutMin=[]  NOutMax=[]  SumOutMin=[]  SumOutMax=[]  SaturationOutMin=[]  SaturationOutMax=[]  PParamMin=[]  PParamMax=[]  IParamMin=[]  IParamMax=[]  DParamMin=[]  DParamMax=[]  NParamMin=[]  NParamMax=[]  KbParamMin=[]  KbParamMax=[]  KtParamMin=[]  KtParamMax=[]  KbOutMin=[]  KbOutMax=[]  KtOutMin=[]  KtOutMax=[]  IntegratorOutMin=[]  IntegratorOutMax=[]  FilterOutMin=[]  FilterOutMax=[]  SumI1OutMin=[]  SumI1OutMax=[]  SumI2OutMin=[]  SumI2OutMax=[]  SumI3OutMin=[]  SumI3OutMax=[]  SumI4OutMin=[]  SumI4OutMax=[]  SumDOutMin=[]  SumDOutMax=[]  DifferentiatorOutMin=[]  DifferentiatorOutMax=[]  FilterDiffOutCoefMin=[]  FilterDiffOutCoefMax=[]  ReciprocalOutMin=[]  ReciprocalOutMax=[]  SumDenOutMin=[]  SumDenOutMax=[]  SumNumOutMin=[]  SumNumOutMax=[]  DivideOutMin=[]  DivideOutMax=[]  UdiffTsProdOutMin=[]  UdiffTsProdOutMax=[]  NTsProdOutMin=[]  NTsProdOutMax=[]  UintegralTsProdOutMin=[]  UintegralTsProdOutMax=[]  UngainTsProdOutMin=[]  UngainTsProdOutMax=[]  ClampingZeroOutDataTypeStr=Inherit: Inherit via back propagation  ClampingZeroOutMin=[]  ClampingZeroOutMax=[]  FilterDenConstantOutDataTypeStr=Inherit: Inherit via back propagation  FilterDenConstantOutMin=[]  FilterDenConstantOutMax=[]  PCopyOutDataTypeStr=Inherit: Inherit via back propagation  PCopyOutMin=[]  PCopyOutMax=[]  NCopyOutDataTypeStr=Inherit: Inherit via back propagation  NCopyOutMin=[]  NCopyOutMax=[]  IntegratorContinuousStateAttributes=''  IntegratorStateMustResolveToSignalObject=off  IntegratorRTWStateStorageClass=Auto  FilterContinuousStateAttributes=''  FilterStateMustResolveToSignalObject=off  FilterRTWStateStorageClass=Auto  ParallelPVariant=InternalParameters  IdealPVariant=Disabled  IVariant=InternalParameters  DVariant=InternalParameters  IntegratorVariant=Continuous  SatVariant=Disabled  AWVariant=Passthrough  PCopyVariant=Disabled  TRVariant=Disabled  FdbkBlocksVariant=Forward  IdealPFdbkVariant=Disabled  SatFdbkVariant=Disabled  DerivativeFilterVariant=ContFilter  NVariant=InternalParameters  NCopyVariant=Disabled  FilterICVariant=InternalICsFilter  IntegratorICVariant=InternalICs  ExternalResetVariant=Disabled  TRSumVariant=Passthrough  SumFdbkVariant=Disabled  SumVariant=Sum_PID  TsampFilterVariant=InternalTs  TsampNgainVariant=Passthrough  TsampIntegralVariant=Passthrough  ExternalSaturationOutDataTypeStr=Inherit: Same as second input
  Sum : Sum  Inputs=|+-
  Sum1 : Sum  Inputs=|+-
  u : Outport
  u1 : Outport  Port=2
  wires:
  Sum1/1 -> PID Controller1/1
  Sum/1 -> PID Controller/1
  PID Controller/1 -> u/1
  PID Controller1/1 -> u1/1
  Input/1 -> Sum/2
  From Workspace/1 -> Sum/1
  From Workspace1/1 -> Sum1/1
  Input1/1 -> Sum1/2

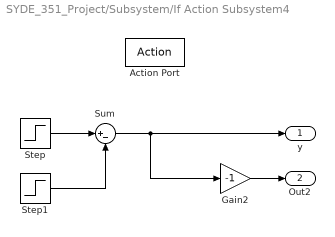
== system SYDE_351_Project/Subsystem/If Action Subsystem4 ==
  Action Port : ActionPort  ActionPortLabel=elseif( (u1 > 15.3583) & (u1 <= 19.3833))
  Gain2 : Gain  Gain=-1
  Step : Step  Time=15.3583  After=1.7  SampleTime=0
  Step1 : Step  Time=16.83  After=1.7  SampleTime=0
  Sum : Sum  Inputs=|+-
  y : Outport
  Out2 : Outport  Port=2
  wires:
  Gain2/1 -> Out2/1
  Sum/1 -> y/1, Gain2/1
  Step/1 -> Sum/1
  Step1/1 -> Sum/2

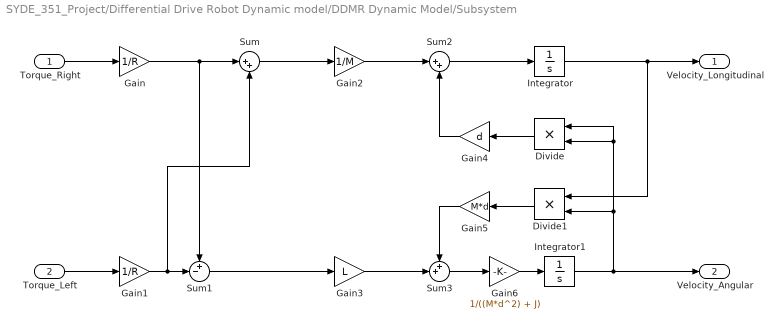
== system SYDE_351_Project/Differential Drive Robot Dynamic model/DDMR Dynamic Model/Subsystem ==
  Torque_Right : Inport
  Torque_Left : Inport  Port=2
  Divide : Product  Inputs=**
  Divide1 : Product  Inputs=**
  Gain : Gain  Gain=1/R
  Gain1 : Gain  Gain=1/R
  Gain2 : Gain  Gain=1/M
  Gain3 : Gain  Gain=L
  Gain4 : Gain  Gain=d
  Gain5 : Gain  Gain=M*d
  Gain6 : Gain  Gain=1/((M*d^2) + J)
  Integrator : Integrator
  Integrator1 : Integrator
  Sum : Sum  Inputs=|++
  Sum1 : Sum  Inputs=+-|
  Sum2 : Sum  Inputs=|++
  Sum3 : Sum  Inputs=++|
  Velocity_Longitudinal : Outport
  Velocity_Angular : Outport  Port=2
  wires:
  Gain5/1 -> Sum3/1
  Divide/1 -> Gain4/1
  Gain3/1 -> Sum3/2
  Torque_Left/1 -> Gain1/1
  Torque_Right/1 -> Gain/1
  Integrator/1 -> Divide1/1, Velocity_Longitudinal/1
  Gain6/1 -> Integrator1/1
  Gain/1 -> Sum1/1, Sum/1
  Gain4/1 -> Sum2/2
  Divide1/1 -> Gain5/1
  Sum/1 -> Gain2/1
  Gain1/1 -> Sum/2, Sum1/2
  Integrator1/1 -> Velocity_Angular/1, Divide1/2, Divide/1, Divide/2
  Gain2/1 -> Sum2/1
  Sum3/1 -> Gain6/1
  Sum1/1 -> Gain3/1
  Sum2/1 -> Integrator/1

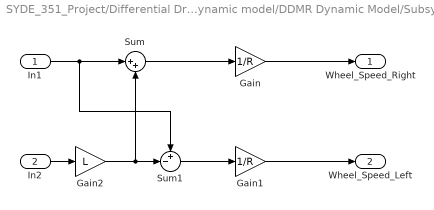
== system SYDE_351_Project/Differential Drive Robot Dynamic model/DDMR Dynamic Model/Subsystem1 ==
  In1 : Inport
  In2 : Inport  Port=2
  Gain : Gain  Gain=1/R
  Gain1 : Gain  Gain=1/R
  Gain2 : Gain  Gain=L
  Sum : Sum  Inputs=|++
  Sum1 : Sum  Inputs=+-|
  Wheel_Speed_Right : Outport
  Wheel_Speed_Left : Outport  Port=2
  wires:
  Sum/1 -> Gain/1
  Sum1/1 -> Gain1/1
  In1/1 -> Sum1/1, Sum/1
  In2/1 -> Gain2/1
  Gain/1 -> Wheel_Speed_Right/1
  Gain1/1 -> Wheel_Speed_Left/1
  Gain2/1 -> Sum/2, Sum1/2

== matlab function SYDE_351_Project/MATLAB Function1 ==
  data: pose input
function drawRobot(pose)

    x = pose(1);
    y = pose(2);
    theta = rad2deg(pose(3));

    radius = 0.25;
    
    theta = theta - 90;
    
    % Get points for circle
    angles = 0:5:360;
    x_c = [cosd(angles)',sind(angles)'];
    x_c = x_c.*radius;

    % Get points for orientation arrow
    p1 = [0.2,-0.4];
    p2 = [0.2,0.4];
    p3 = [0.6,0.4];
    p4 = [0,1];
    inv_x = [-1,1];
    x_a = [p1;p2;p3;p4;inv_x.*p3;inv_x.*p2;inv_x.*p1;p1];
    x_a = x_a.*radius;

    % Rotation matrix for theta
    rot_trans = [cosd(theta), -sind(theta), x; sind(theta), cosd(theta), y; 0 0 1];
    
    % Apply rotation and translation to points
    x_c = rot_trans*[x_c,ones(size(x_c(:,1)))]';
    x_a = rot_trans*[x_a,ones(size(x_a(:,1)))]';
    x_c = x_c(1:2,:)';
    x_a = x_a(1:2,:)';
    
    plot(x_c(:,1),x_c(:,2),'blue'); hold on;
    plot(x_a(:,1),x_a(:,2),'red');

end
